simulink model "rigid_body_model"  (R2016a)
settings: Solver=VariableStepAuto  StartTime=0.0  StopTime=20  RelTol=1e-3
undefined symbols (not defined in the file): g, gammaC, h, IB, l, lcm, ld, m, omega0, p0, q0, r, v0, w
libraries: aerolibutil x1
settings Model: Creator=mgreiff  LastModifiedBy=mgreiff

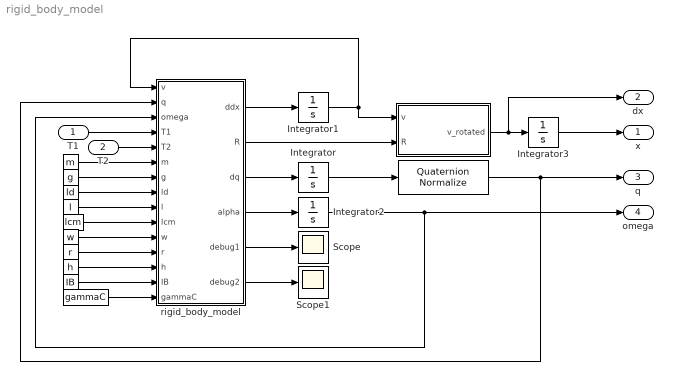
== system rigid_body_model ==
  T1 : Inport  PortDimensions=3
  T2 : Inport  Port=2  PortDimensions=3
  " " : Constant  Value=ld
  "  " : Constant  Value=m
  "   " : Constant  Value=g
  "    " : Constant  Value=l
  "     " : Constant  Value=lcm
  "      " : Constant  Value=w
  "       " : Constant  Value=r
  "        " : Constant  Value=h
  "         " : Constant  Value=IB
  "           " : Constant  Value=gammaC
  "             " : MATLAB Function  TreatAsAtomicUnit=on
  "                    " : aerolibutil/Quaternion Normalize
  Integrator : Integrator  InitialCondition=q0
  Integrator1 : Integrator  InitialCondition=v0
  Integrator2 : Integrator  InitialCondition=omega0
  Integrator3 : Integrator  InitialCondition=p0
  Scope : Scope
  Scope1 : Scope
  rigid_body_model : MATLAB Function  TreatAsAtomicUnit=on
  x : Outport  PortDimensions=3
  dx : Outport  Port=2  PortDimensions=3
  q : Outport  Port=3  PortDimensions=4
  omega : Outport  Port=4  PortDimensions=3
  wires:
  rigid_body_model/4(alpha) -> Integrator2/1
  rigid_body_model/1(ddx) -> Integrator1/1
  rigid_body_model/3(dq) -> Integrator/1
  T1/1 -> rigid_body_model/4(T1)
  T2/1 -> rigid_body_model/5(T2)
  " "/1 -> rigid_body_model/8(ld)
  "  "/1 -> rigid_body_model/6(m)
  "   "/1 -> rigid_body_model/7(g)
  "    "/1 -> rigid_body_model/9(l)
  "     "/1 -> rigid_body_model/10(lcm)
  "      "/1 -> rigid_body_model/11(w)
  "       "/1 -> rigid_body_model/12(r)
  "        "/1 -> rigid_body_model/13(h)
  Integrator1/1 -> rigid_body_model/1(v), "             "/1(v)
  Integrator3/1 -> x/1
  "         "/1 -> rigid_body_model/14(IB)
  rigid_body_model/2(R) -> "             "/2(R)
  Integrator2/1 -> rigid_body_model/3(omega), omega/1
  Integrator/1 -> "                    "/1
  "           "/1 -> rigid_body_model/15(gammaC)
  "                    "/1 -> rigid_body_model/2(q), q/1
  rigid_body_model/5(debug1) -> Scope/1
  rigid_body_model/6(debug2) -> Scope1/1
  "             "/1(v_rotated) -> dx/1, Integrator3/1

== matlab function rigid_body_model/              ==
  data: v input; R input; v_rotated output
function v_rotated = rotateVelocity(v, R)
%#codegen
v_rotated = R*v;

== matlab function rigid_body_model/rigid_body_model ==
  data: v input; q input; ddx output; R output; dq output; omega input; alpha output; T1 input; T2 input; m input; g input; ld input; l input; lcm input; w input; r input; h input; IB input; gammaC input; debug1 output; debug2 output
function [ddx, R, dq, alpha, debug1, debug2] = rigid_body(v, q, omega, T1, T2, m, g, ld, l, lcm, w, r, h, IB, gammaC)
% Sets upp the system B = AX + C

% System vectors
dcm = [lcm, 0, 0]';
d1 = [0, -w, 0]';
d2 = [0,  w, 0]';
d3 = [l,  w, 0]';
d4 = [l, -w, 0]';
qw = q(1);
qx = q(2);
qy = q(3);
qz = q(4);
qv = q(2:4);

% Matrix operators
I3     = eye(3);
Z3     = zeros(3);
Scm    = get_skew_symmetric_operator(dcm);
Somega = get_skew_symmetric_operator(omega);
S1     = get_skew_symmetric_operator(d1);
S2     = get_skew_symmetric_operator(d2);
S3     = get_skew_symmetric_operator(d3);
S4     = get_skew_symmetric_operator(d4);
Squat  = get_skew_symmetric_operator(qv);

% Friction model
F1 = -gammaC.*(-cross(d1, omega) + v);
F2 = -gammaC.*(-cross(d2, omega) + v);
F3 = -gammaC.*(-cross(d3, omega) + v);
F4 = -gammaC.*(-cross(d4, omega) + v);
F1(3) = 0;
F2(3) = 0;
F3(3) = 0;
F4(3) = 0;

% Parametrizes rotation matrix
R = [qw^2+qx^2-qy^2-qz^2, 2*(qx*qy-qw*qz)    , 2*(qx*qz+qw*qy);
     2*(qx*qy+qw*qz)    , qw^2-qx^2+qy^2-qz^2, 2*(qy*qz-qw*qx);
     2*(qx*qz-qw*qy)    , 2*(qy*qz+qw*qx)    , qw^2-qx^2-qy^2+qz^2];

% Sets up A
model = 1; 
switch model
    case 1
        A = [m.*I3, Z3;...
             Z3   , IB];
    case 2
        A = [m.*I3 , -m.*Scm;...
             m.*Scm, IB - m.*Scm*Scm];
end

% Sets up B
Forces = T1 + T2 + F1 + F2 + F3 + F4;
Torques = S1*(T1 + F1) + S2*(T2 + F2) + S3*F3 + S4*F4;
B = [Forces;...
     Torques];

% Sets up C
switch model
    case 1
        C = [zeros(3,1);...
             Somega * (IB*omega)];
    case 2
        C = [m.* Somega * Somega * dcm;...
             Somega * (IB - m.*Scm*Scm) * omega];
end
% Solves system
X = A\(B - C);

% Externalizes state
dq = 0.5.*(eye(4).*qw  + [0, -qv';qv, Squat])*[0; omega];
alpha = X(4:6);
ddx = X(1:3);

debug1 = R*X(1:3);
debug2 = R'*[1;0;0];
end

function [S] = get_skew_symmetric_operator(u)
S = [0   , -u(3), u(2);...
     u(3), 0   , -u(1);...
     -u(2), u(1), 0   ];
end
